simulink model "FermentationV3"  (R2023b)
settings: Solver=FixedStepAuto  StartTime=3220  StopTime=16770  FixedStep=1  RelTol=1e-3
values from neighbouring files (symbols this model uses):
  sug_current = sug_init    (= 1011.832)    [init_4_sim.m]    (also in init_sim2.m; init_sim_suggarferm.m)
  sug_init = 1011.832    [init_4_sim.m]    (also in init_sim.m = 1011; init_sim2.m; init_sim_suggarferm.m)
  t_step = 1    [init_4_sim.m]    (also in init_sim2.m; init_sim_suggarferm.m; startingThermodynamics.m)
  temp = 296    [init_4_sim.m]    (also in init_sim.m = 298.15; init_sim2.m; init_sim_suggarferm.m)
  volume = 25    [init_4_sim.m]    (also in init_sim.m; init_sim2.m; init_sim_suggarferm.m)
  yeast_gram = 11    [init_4_sim.m]    (also in init_sim2.m; init_sim_suggarferm.m)
settings Model: PacingRate=10  Creator=20181234  LastModifiedBy=20181234

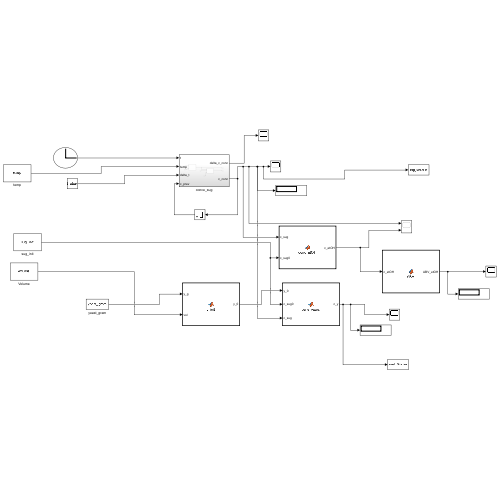
[thumbnail: Simulink's stored preview of the top-level diagram]
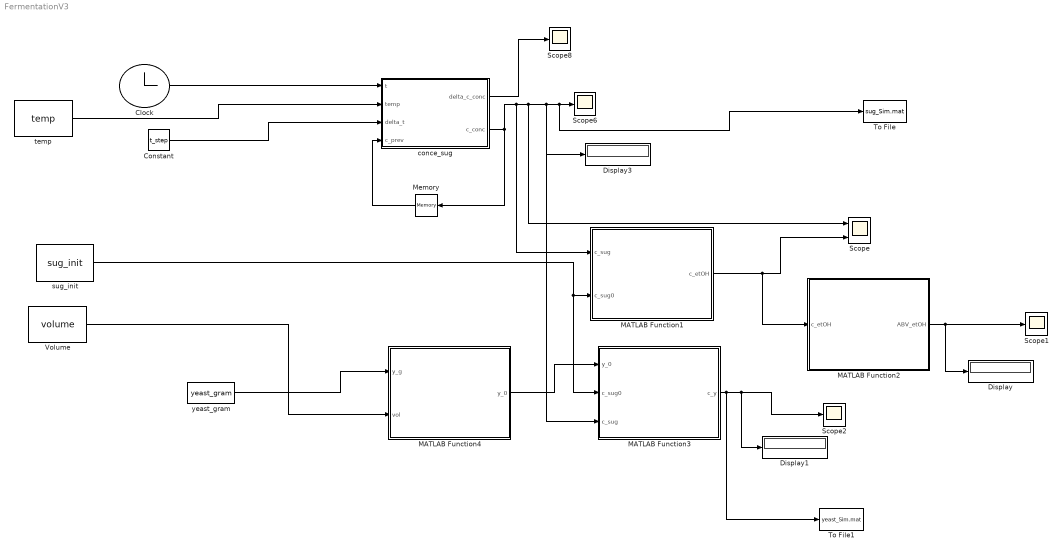
== system FermentationV3 ==
  Clock : Clock
  Constant : Constant  Value=t_step
  Display : Display
  Display1 : Display
  Display3 : Display
  MATLAB Function1 : MATLAB Function  TreatAsAtomicUnit=on
  MATLAB Function2 : MATLAB Function  TreatAsAtomicUnit=on
  MATLAB Function3 : MATLAB Function  TreatAsAtomicUnit=on
  MATLAB Function4 : MATLAB Function  TreatAsAtomicUnit=on
  Memory : Memory  InitialCondition=sug_current
  Scope : Scope  NumInputPorts=2
  Scope{1..2,6,8} (4 alike) : Scope
  To File : ToFile  Filename=sug_Sim.mat  MatrixName=sug_conc
  To File1 : ToFile  Filename=yeast_Sim.mat  MatrixName=yeast
      settings: Decimation=2
  Volume : Constant  Value=volume
  conce_sug : Subsystem
  sug_init : Constant  Value=sug_init
  temp : Constant  Value=temp
  yeast_gram : Constant  Value=yeast_gram
  wires:
  Clock/1 -> conce_sug/1(t)
  temp/1 -> conce_sug/2(temp)
  sug_init/1 -> MATLAB Function3/2(c_sug0), MATLAB Function1/2(c_sug0)
  MATLAB Function1/1(c_etOH) -> MATLAB Function2/1(c_etOH), Scope/2
  MATLAB Function2/1(ABV_etOH) -> Display/1, Scope1/1
  MATLAB Function3/1(c_y) -> To File1/1, Display1/1, Scope2/1
  yeast_gram/1 -> MATLAB Function4/1(y_g)
  Volume/1 -> MATLAB Function4/2(vol)
  MATLAB Function4/1(y_0) -> MATLAB Function3/1(y_0)
  Memory/1 -> conce_sug/4(c_prev)
  conce_sug/2(c_conc) -> Memory/1, MATLAB Function1/1(c_sug), Scope/1, MATLAB Function3/3(c_sug), Display3/1, To File/1, Scope6/1
  Constant/1 -> conce_sug/3(delta_t)
  conce_sug/1(delta_c_conc) -> Scope8/1

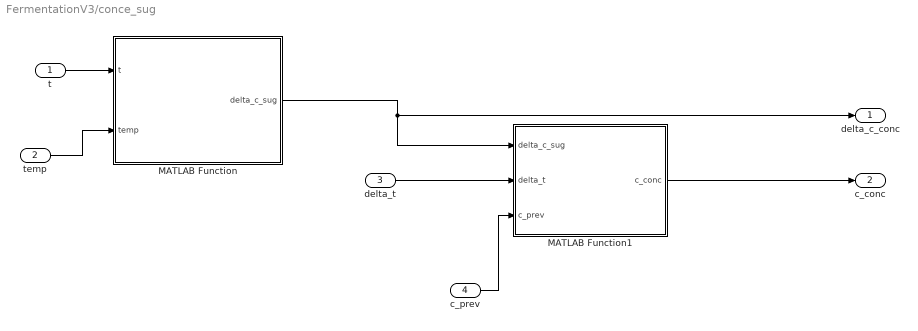
== system FermentationV3/conce_sug ==
  t : Inport
  temp : Inport  Port=2
  delta_t : Inport  Port=3
  c_prev : Inport  Port=4
  MATLAB Function : MATLAB Function  TreatAsAtomicUnit=on
  MATLAB Function1 : MATLAB Function  TreatAsAtomicUnit=on
  delta_c_conc : Outport
  c_conc : Outport  Port=2
  wires:
  MATLAB Function/1(delta_c_sug) -> delta_c_conc/1, MATLAB Function1/1(delta_c_sug)
  MATLAB Function1/1(c_conc) -> c_conc/1
  t/1 -> MATLAB Function/1(t)
  temp/1 -> MATLAB Function/2(temp)
  delta_t/1 -> MATLAB Function1/2(delta_t)
  c_prev/1 -> MATLAB Function1/3(c_prev)

== matlab function FermentationV3/MATLAB Function1 ==
  data: c_sug input; c_etOH output; c_sug0 input
function c_etOH = conc_etOH(c_sug,c_sug0)
%stequimetry
st= 1.503;
%st= 1.5075;



c_etOH = (c_sug0-c_sug)*st;

== matlab function FermentationV3/MATLAB Function2 ==
  data: c_etOH input; ABV_etOH output
function ABV_etOH = ABV(c_etOH)
%stequimetry
MW_etOH = 46;%mol/g
density_etOH = 0.789; %g/ml




ABV_etOH = c_etOH*(MW_etOH/density_etOH)/1000^2*100;

== matlab function FermentationV3/MATLAB Function3 ==
  data: y_0 input; c_sug0 input; c_sug input; c_y output
function c_y = conc_yeast(y_0,c_sug0,c_sug)
%stequimetry
Y_trans = 0.1;
MW_sug = 180.16; %g/mol
MW_y = 24; %g/mol



c_y = (c_sug0-c_sug)*(MW_sug/MW_y)*Y_trans+y_0;

== matlab function FermentationV3/MATLAB Function4 ==
  data: y_g input; vol input; y_0 output
function y_0 = y_init(y_g,vol)

MW_y = 24; %g/mol


y_0 = (y_g/(vol*1000))/MW_y;

== matlab function FermentationV3/conce_sug/MATLAB Function ==
  data: t input; delta_c_sug output; temp input
function delta_c_sug = dela_conc_sug(t,temp)
A = 1.24503386e-22;
E = -9.35902242e4;
m = -0.000132816;
b = -0.058764065;
R = 8.314; %j/molK

c1=A*exp(-E/(R*temp));
c2=m*temp + b;

delta_c_sug = 2*c1*t+c2;
if delta_c_sug >= 0
    delta_c_sug = 0;
end

== matlab function FermentationV3/conce_sug/MATLAB Function1 ==
  data: delta_c_sug input; c_conc output; delta_t input; c_prev input
function c_conc = c_conc_func(delta_c_sug, delta_t,c_prev)

c_conc = c_prev + delta_t*delta_c_sug;
